simulink model "cartesian_regulation_ctrl"  (R2025b)
settings: Solver=VariableStepAuto  StartTime=0.0  StopTime=10  RelTol=1e-3
libraries: robotmobilelib x1
settings Model: Creator=alessandrochinello  LastModifiedBy=matti

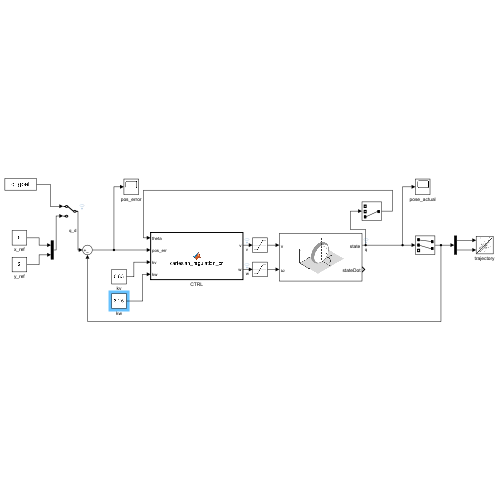
[thumbnail: Simulink's stored preview of the top-level diagram]
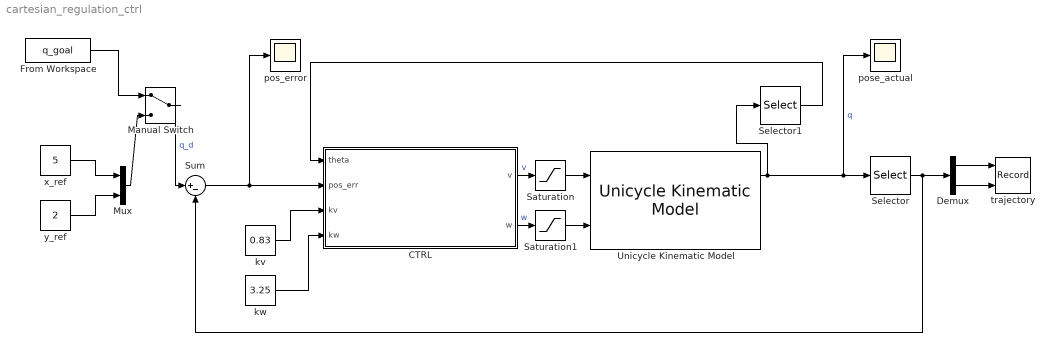
== system cartesian_regulation_ctrl ==
  CTRL : MATLAB Function  TreatAsAtomicUnit=on
  Demux : Demux  Outputs=2
  From Workspace : FromWorkspace  VariableName=q_goal
  Manual Switch : ManualSwitch
  Mux : Mux  Inputs=2
  Saturation : Saturate  UpperLimit=1  LowerLimit=-1
  Saturation1 : Saturate  UpperLimit=pi/2  LowerLimit=-pi/2
  Selector : Selector  InputPortWidth=3  IndexOptions=Index vector (dialog)  Indices=[1 2]  OutputSizes=1
  Selector1 : Selector  InputPortWidth=3  IndexOptions=Index vector (dialog)  Indices=[3]  OutputSizes=1
  Sum : Sum  Inputs=|+-
  Unicycle Kinematic Model : robotmobilelib/Unicycle Kinematic Model  VehicleInputs=Vehicle Speed & Heading Angular Velocity  WheelRadius=0.1  WheelSpeedRange=[-Inf Inf]  InitialState=q0_reg  SimulateUsing=Interpreted execution
  kv : Constant  Value=0.83
  kw : Constant  Value=3.25
  pos_error : Scope
      settings: ActiveDisplayYMinimum=-256.17429974027243  ActiveDisplayYMaximum=116.62668553365748
  pose_actual : Scope
      settings: ActiveDisplayYMinimum=-37.155041353571882  ActiveDisplayYMaximum=8.5892802665132866
  trajectory : Record  NumPorts=2.0  FileSettingsInternal="{\"entries\":[{\"content\":{\"excelSettings\":{\"content\":{},\"type\":\"Streamout.ExcelSettings\"},\"parquetSettings\":{\"content\":{},\"type\":\"Streamout.ParquetSettings\"}},\"type\":\"Streamout.FileSettingStorage\",\"uuid\":\"\"}],\"packageUris\":[\"http:\\/\\/schema.mathworks.com\\/mf0\\/streamout_blocks\\/R2020a\"],\"version\":\"1.0\"}"  FrameSettings=[0, 0]  Layout=[1 1]  SignalsInternal="{\"entries\":[{\"content\":{\"signals\":[{\"content\":{\"blockPath\":[],\"dimensions\":[1],\"domain\":\"\",\"lineColor\":\"#a2142f\",\"plots\":[ 1 ],\"port\":1,\"signalID\":1,\"signalName\":\"Demux:1\"},\"type\":\"RecordBlkView.Signal\",\"uuid\":\"\"},{\"content\":{\"blockPath\":[],\"dimensions\":[1],\"domain\":\"\",\"lineColor\":\"#139fff\",\"plots\":[ 1 ],\"port\":2,\"signalID\":2,\"signalName\":\"Demux:2\"},\"type\":\"RecordBlkView.Signal\",\"uuid\":\"\"}]},\"type\":\"RecordBlkView.InputSignals\",\"uuid\":\"\"}],\"packageUris\":[\"http:\\/\\/schema.mathworks.com\\/mf0\\/streamout_blocks\\/R2020a\"],\"version\":\"1.0\"}"  VisualizationBindings="{\"xyplotplugin\":{\"info\":[{\"series\":[{\"bindingParametersList\":[{\"parameter\":\"X-Axis\",\"signalID\":1,\"signalName\":\"Demux:1\"},{\"parameter\":\"Y-Axis\",\"signalID\":2,\"signalName\":\"Demux:2\"}],\"seriesID\":0}],\"subplotID\":1}]}}"  CompatibilityTag=XY
  x_ref : Constant  Value=5
  y_ref : Constant  Value=2
  wires:
  CTRL/2(w) -> Saturation1/1  "w"
  CTRL/1(v) -> Saturation/1  "v"
  x_ref/1 -> Mux/1
  y_ref/1 -> Mux/2
  Unicycle Kinematic Model/1 -> pose_actual/1, Selector/1, Selector1/1  "q"
  kv/1 -> CTRL/3(kv)
  kw/1 -> CTRL/4(kw)
  Sum/1 -> CTRL/2(pos_err), pos_error/1
  Demux/1 -> trajectory/1
  Demux/2 -> trajectory/2
  Selector/1 -> Demux/1, Sum/2
  Selector1/1 -> CTRL/1(theta)
  From Workspace/1 -> Manual Switch/1
  Mux/1 -> Manual Switch/2
  Manual Switch/1 -> Sum/1  "q_d"
  Saturation/1 -> Unicycle Kinematic Model/1
  Saturation1/1 -> Unicycle Kinematic Model/2

== matlab function cartesian_regulation_ctrl/CTRL ==
  data: theta input; pos_err input; v output; w output; kv input; kw input
function [v, w] = cartesian_regulation_crl(theta, pos_err, kv, kw)

n = [cos(theta); sin(theta)];
target_angle = atan2(pos_err(2), pos_err(1));
gamma = wrapToPi(target_angle - theta);

v = kv * dot(pos_err, n);
w = kw * gamma;

end
